simulink model "MotionGeneration"  (R2023a)
settings: Solver=VariableStepAuto  StartTime=0.0  StopTime=20
values from neighbouring files (symbols this model uses):
  C_D = 24/Re*(1+0.15*(Re)^(1/2)+0.017*Re) - (0.208/(1+10^4*Re^(-0.5)))    (= 0.446659281404)    [Param.m]
  C_m = 0.5    [Param.m]
  C_w = 3    [Param.m]
  d = 0.01    [Param.m]
  I = 2/5*M*R^2    (= 1.2723450247e-06)    [Param.m]
  M = 4/3*pi*R^3*p    (= 0.0141371669412)    [Param.m]
  p = 1000    [Param.m]
  R = 0.015    [Param.m]
libraries: slpidlib x2
settings Model: Creator=vader04  LastModifiedBy=vader04

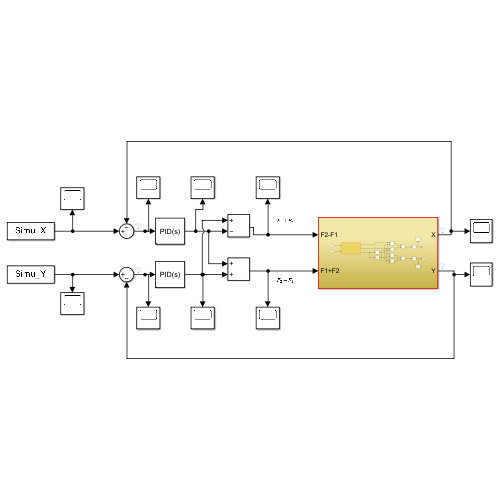
[thumbnail: Simulink's stored preview of the top-level diagram]
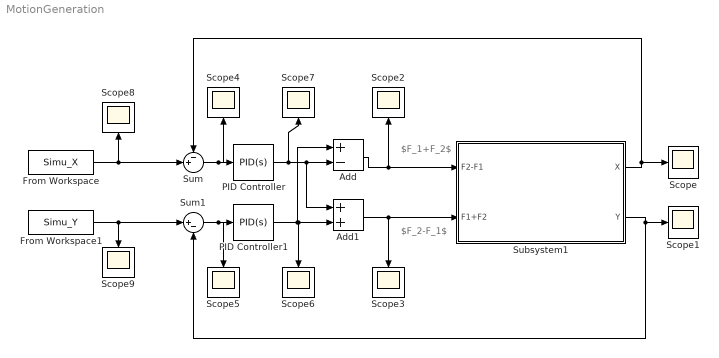
== system MotionGeneration ==
  note: $F_1+F_2$
  note: $F_2-F_1$
  Add : Sum  Inputs=+-
  Add1 : Sum
  From Workspace : FromWorkspace  VariableName=Simu_X
  From Workspace1 : FromWorkspace  VariableName=Simu_Y
  PID Controller : slpidlib/PID Controller  Controller=PID  Form=Parallel  TimeDomain=Continuous-time  UseExternalTs=off  SampleTime=-1  IntegratorMethod=Forward Euler  FilterMethod=Forward Euler  ControllerParametersSource=internal  P=0.8  I=0.5  UseKiTs=off  D=20  N=4.19588623240931  UseFilter=on  TunerSelectOption=Transfer Function Based (PID Tuner App)  InitialConditionSource=internal  InitialConditionForIntegrator=0  InitialConditionForFilter=0  DifferentiatorICPrevScaledInput=0  ExternalReset=none  TrackingMode=off  Kt=1  LimitOutput=off  SatLimitsSource=internal  UpperSaturationLimit=inf  LowerSaturationLimit=-inf  LinearizeAsGain=on  AntiWindupMode=none  Kb=1  LimitIntegrator=off  UpperIntegratorSaturationLimit=inf  LowerIntegratorSaturationLimit=-inf  POutMin=[]  POutMax=[]  IOutMin=[]  IOutMax=[]  DOutMin=[]  DOutMax=[]  NOutMin=[]  NOutMax=[]  SumOutMin=[]  SumOutMax=[]  SaturationOutMin=[]  SaturationOutMax=[]  PParamMin=[]  PParamMax=[]  IParamMin=[]  IParamMax=[]  DParamMin=[]  DParamMax=[]  NParamMin=[]  NParamMax=[]  KbParamMin=[]  KbParamMax=[]  KtParamMin=[]  KtParamMax=[]  KbOutMin=[]  KbOutMax=[]  KtOutMin=[]  KtOutMax=[]  IntegratorOutMin=[]  IntegratorOutMax=[]  FilterOutMin=[]  FilterOutMax=[]  SumI1OutMin=[]  SumI1OutMax=[]  SumI2OutMin=[]  SumI2OutMax=[]  SumI3OutMin=[]  SumI3OutMax=[]  SumI4OutMin=[]  SumI4OutMax=[]  SumDOutMin=[]  SumDOutMax=[]  DifferentiatorOutMin=[]  DifferentiatorOutMax=[]  FilterDiffOutCoefMin=[]  FilterDiffOutCoefMax=[]  ReciprocalOutMin=[]  ReciprocalOutMax=[]  SumDenOutMin=[]  SumDenOutMax=[]  SumNumOutMin=[]  SumNumOutMax=[]  DivideOutMin=[]  DivideOutMax=[]  UdiffTsProdOutMin=[]  UdiffTsProdOutMax=[]  NTsProdOutMin=[]  NTsProdOutMax=[]  UintegralTsProdOutMin=[]  UintegralTsProdOutMax=[]  UngainTsProdOutMin=[]  UngainTsProdOutMax=[]  ClampingZeroOutDataTypeStr=Inherit: Inherit via back propagation  ClampingZeroOutMin=[]  ClampingZeroOutMax=[]  FilterDenConstantOutDataTypeStr=Inherit: Inherit via back propagation  FilterDenConstantOutMin=[]  FilterDenConstantOutMax=[]  PCopyOutDataTypeStr=Inherit: Inherit via back propagation  PCopyOutMin=[]  PCopyOutMax=[]  NCopyOutDataTypeStr=Inherit: Inherit via back propagation  NCopyOutMin=[]  NCopyOutMax=[]  IntegratorContinuousStateAttributes=''  IntegratorStateMustResolveToSignalObject=off  IntegratorRTWStateStorageClass=Auto  FilterContinuousStateAttributes=''  FilterStateMustResolveToSignalObject=off  FilterRTWStateStorageClass=Auto  ParallelPVariant=InternalParameters  IdealPVariant=Disabled  IVariant=InternalParameters  DVariant=InternalParameters  IntegratorVariant=Continuous  SatVariant=Disabled  AWVariant=Passthrough  PCopyVariant=Disabled  TRVariant=Disabled  FdbkBlocksVariant=Forward  IdealPFdbkVariant=Disabled  SatFdbkVariant=Disabled  DerivativeFilterVariant=ContFilter  NVariant=InternalParameters  NCopyVariant=Disabled  FilterICVariant=InternalICsFilter  IntegratorICVariant=InternalICs  ExternalResetVariant=Disabled  TRSumVariant=Passthrough  SumFdbkVariant=Disabled  SumVariant=Sum_PID  TsampFilterVariant=InternalTs  TsampNgainVariant=Passthrough  TsampIntegralVariant=Disabled_SignalSpec  ExternalSaturationOutDataTypeStr=Inherit: Same as second input
  PID Controller1 : slpidlib/PID Controller  Controller=PID  Form=Parallel  TimeDomain=Continuous-time  UseExternalTs=off  SampleTime=-1  IntegratorMethod=Forward Euler  FilterMethod=Forward Euler  ControllerParametersSource=internal  P=0.8  I=0.5  UseKiTs=off  D=20  N=4.19588623240931  UseFilter=on  TunerSelectOption=Transfer Function Based (PID Tuner App)  InitialConditionSource=internal  InitialConditionForIntegrator=0  InitialConditionForFilter=0  DifferentiatorICPrevScaledInput=0  ExternalReset=none  TrackingMode=off  Kt=1  LimitOutput=off  SatLimitsSource=internal  UpperSaturationLimit=inf  LowerSaturationLimit=-inf  LinearizeAsGain=on  AntiWindupMode=none  Kb=1  LimitIntegrator=off  UpperIntegratorSaturationLimit=inf  LowerIntegratorSaturationLimit=-inf  POutMin=[]  POutMax=[]  IOutMin=[]  IOutMax=[]  DOutMin=[]  DOutMax=[]  NOutMin=[]  NOutMax=[]  SumOutMin=[]  SumOutMax=[]  SaturationOutMin=[]  SaturationOutMax=[]  PParamMin=[]  PParamMax=[]  IParamMin=[]  IParamMax=[]  DParamMin=[]  DParamMax=[]  NParamMin=[]  NParamMax=[]  KbParamMin=[]  KbParamMax=[]  KtParamMin=[]  KtParamMax=[]  KbOutMin=[]  KbOutMax=[]  KtOutMin=[]  KtOutMax=[]  IntegratorOutMin=[]  IntegratorOutMax=[]  FilterOutMin=[]  FilterOutMax=[]  SumI1OutMin=[]  SumI1OutMax=[]  SumI2OutMin=[]  SumI2OutMax=[]  SumI3OutMin=[]  SumI3OutMax=[]  SumI4OutMin=[]  SumI4OutMax=[]  SumDOutMin=[]  SumDOutMax=[]  DifferentiatorOutMin=[]  DifferentiatorOutMax=[]  FilterDiffOutCoefMin=[]  FilterDiffOutCoefMax=[]  ReciprocalOutMin=[]  ReciprocalOutMax=[]  SumDenOutMin=[]  SumDenOutMax=[]  SumNumOutMin=[]  SumNumOutMax=[]  DivideOutMin=[]  DivideOutMax=[]  UdiffTsProdOutMin=[]  UdiffTsProdOutMax=[]  NTsProdOutMin=[]  NTsProdOutMax=[]  UintegralTsProdOutMin=[]  UintegralTsProdOutMax=[]  UngainTsProdOutMin=[]  UngainTsProdOutMax=[]  ClampingZeroOutDataTypeStr=Inherit: Inherit via back propagation  ClampingZeroOutMin=[]  ClampingZeroOutMax=[]  FilterDenConstantOutDataTypeStr=Inherit: Inherit via back propagation  FilterDenConstantOutMin=[]  FilterDenConstantOutMax=[]  PCopyOutDataTypeStr=Inherit: Inherit via back propagation  PCopyOutMin=[]  PCopyOutMax=[]  NCopyOutDataTypeStr=Inherit: Inherit via back propagation  NCopyOutMin=[]  NCopyOutMax=[]  IntegratorContinuousStateAttributes=''  IntegratorStateMustResolveToSignalObject=off  IntegratorRTWStateStorageClass=Auto  FilterContinuousStateAttributes=''  FilterStateMustResolveToSignalObject=off  FilterRTWStateStorageClass=Auto  ParallelPVariant=InternalParameters  IdealPVariant=Disabled  IVariant=InternalParameters  DVariant=InternalParameters  IntegratorVariant=Continuous  SatVariant=Disabled  AWVariant=Passthrough  PCopyVariant=Disabled  TRVariant=Disabled  FdbkBlocksVariant=Forward  IdealPFdbkVariant=Disabled  SatFdbkVariant=Disabled  DerivativeFilterVariant=ContFilter  NVariant=InternalParameters  NCopyVariant=Disabled  FilterICVariant=InternalICsFilter  IntegratorICVariant=InternalICs  ExternalResetVariant=Disabled  TRSumVariant=Passthrough  SumFdbkVariant=Disabled  SumVariant=Sum_PID  TsampFilterVariant=InternalTs  TsampNgainVariant=Passthrough  TsampIntegralVariant=Disabled_SignalSpec  ExternalSaturationOutDataTypeStr=Inherit: Same as second input
  Scope{,1..9} (10 alike) : Scope
  Subsystem1 : Subsystem
  Sum : Sum  Inputs=-+|
  Sum1 : Sum  Inputs=|+-
  wires:
  From Workspace/1 -> Scope8/1, Sum/2
  Subsystem1/1(X) -> Sum/1, Scope/1
  From Workspace1/1 -> Scope9/1, Sum1/1
  Subsystem1/2(Y) -> Sum1/2, Scope1/1
  Add1/1 -> Scope3/1, Subsystem1/2(F1+F2)
  Sum/1 -> Scope4/1, PID Controller/1
  Sum1/1 -> Scope5/1, PID Controller1/1
  Add/1 -> Subsystem1/1(F2-F1), Scope2/1
  PID Controller/1 -> Add1/1, Add/2, Scope7/1
  PID Controller1/1 -> Add/1, Add1/2, Scope6/1

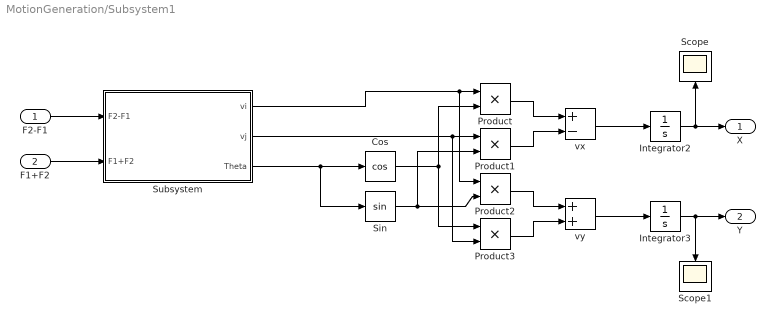
== system MotionGeneration/Subsystem1 ==
  F2-F1 : Inport
  F1+F2 : Inport  Port=2
  Cos : Trigonometry  Operator=cos
  Integrator2 : Integrator
  Integrator3 : Integrator
  Product{,1..3} (4 alike) : Product
  Scope : Scope
  Scope1 : Scope
  Sin : Trigonometry
  Subsystem : Subsystem
  vx : Sum  Inputs=+-
  vy : Sum
  X : Outport
  Y : Outport  Port=2
  wires:
  F1+F2/1 -> Subsystem/2(F1+F2)
  Integrator3/1 -> Y/1, Scope1/1
  Subsystem/2(vj) -> Product3/2, Product1/1
  vy/1 -> Integrator3/1
  Cos/1 -> Product3/1, Product/2
  Product1/1 -> vx/2
  Product3/1 -> vy/2
  Subsystem/1(vi) -> Product2/1, Product/1
  Integrator2/1 -> X/1, Scope/1
  Subsystem/3(Theta) -> Sin/1, Cos/1
  Sin/1 -> Product2/2, Product1/2
  Product/1 -> vx/1
  Product2/1 -> vy/1
  vx/1 -> Integrator2/1
  F2-F1/1 -> Subsystem/1(F2-F1)

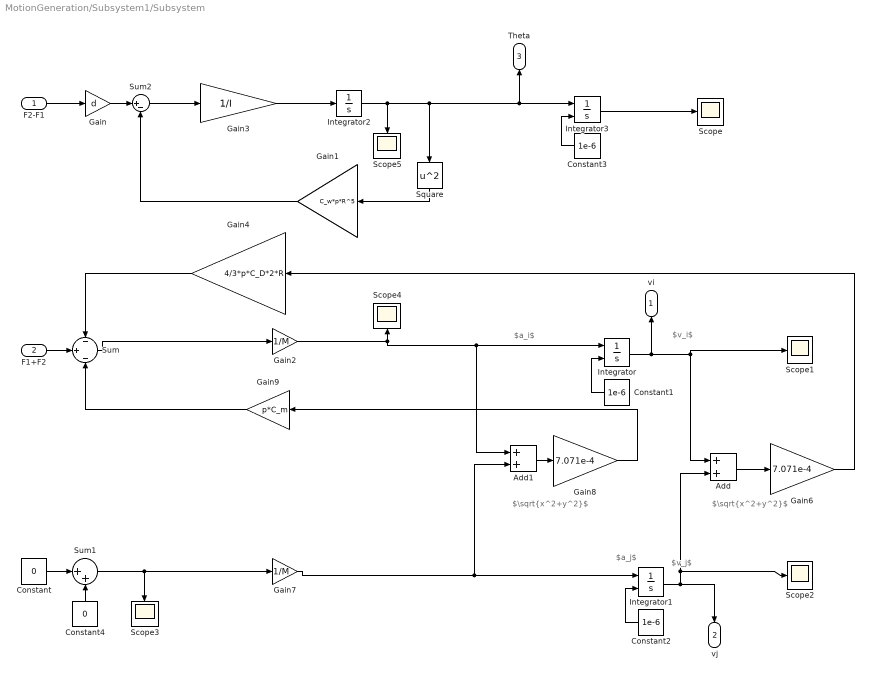
== system MotionGeneration/Subsystem1/Subsystem ==
  note: $\sqrt{x^2+y^2}$
  note: $v_j$
  note: $\sqrt{x^2+y^2}$
  note: $a_i$
  note: $v_i$
  note: $a_j$
  F2-F1 : Inport
  F1+F2 : Inport  Port=2
  Add : Sum
  Add1 : Sum
  Constant : Constant  Value=0
  Constant1 : Constant  Value=1e-6
  Constant2 : Constant  Value=1e-6
  Constant3 : Constant  Value=1e-6
  Constant4 : Constant  Value=0
  Gain : Gain  Gain=d
  Gain1 : Gain  Gain=C_w*p*R^5
  Gain2 : Gain  Gain=1/M
  Gain3 : Gain  Gain=1/I
  Gain4 : Gain  Gain=4/3*p*C_D*2*R
  Gain6 : Gain  Gain=7.071e-4
  Gain7 : Gain  Gain=1/M
  Gain8 : Gain  Gain=7.071e-4
  Gain9 : Gain  Gain=p*C_m
  Integrator : Integrator  InitialConditionSource=external
  Integrator1 : Integrator  InitialConditionSource=external
  Integrator2 : Integrator
  Integrator3 : Integrator  InitialConditionSource=external
  Scope{,1..5} (6 alike) : Scope
  Square : Math  Operator=square
  Sum : Sum  Inputs=-|+|-
  Sum1 : Sum  Inputs=|++
  Sum2 : Sum  Inputs=|+-
  vi : Outport
  vj : Outport  Port=2
  Theta : Outport  Port=3
  wires:
  Gain6/1 -> Gain4/1
  Gain7/1 -> Integrator1/1, Add1/2
  Gain2/1 -> Add1/1, Integrator/1, Scope4/1
  Gain/1 -> Sum2/1
  F1+F2/1 -> Sum/2
  Gain8/1 -> Gain9/1
  Integrator3/1 -> Scope/1
  Integrator/1 -> vi/1, Scope1/1, Add/1
  F2-F1/1 -> Gain/1
  Integrator2/1 -> Scope5/1, Square/1, Theta/1, Integrator3/1
  Constant/1 -> Sum1/1
  Gain1/1 -> Sum2/2
  Constant3/1 -> Integrator3/2
  Constant4/1 -> Sum1/2
  Constant2/1 -> Integrator1/2
  Gain9/1 -> Sum/3
  Gain3/1 -> Integrator2/1
  Integrator1/1 -> vj/1, Scope2/1, Add/2
  Sum1/1 -> Scope3/1, Gain7/1
  Sum/1 -> Gain2/1
  Square/1 -> Gain1/1
  Gain4/1 -> Sum/1
  Add1/1 -> Gain8/1
  Sum2/1 -> Gain3/1
  Add/1 -> Gain6/1
  Constant1/1 -> Integrator/2
